simulink model "Didou_Telemetry"  (R2020a)
settings: Solver=FixedStepAuto  StartTime=0.0  StopTime=inf  RelTol=1e-3
libraries: robotlib x9
settings Model: SimulationMode=accelerator  Creator=alexemdesgagne  LastModifiedBy=alexemdesgagne
settings OptimizationCC: EnhancedBackFolding=on  PassReuseOutputArgsAs=Individual arguments  ZeroExternalMemoryAtStartup=off  ZeroInternalMemoryAtStartup=off  MaxStackSize=64  OptimizeBlockOrder=speed  DifferentSizesBufferReuse=on  OptimizationCustomize=off  EfficientTunableParamExpr=on
settings DebuggingCC: ParameterTunabilityLossMsg=error
settings HardwareCC: ProdBitPerPointer=32  ProdBitPerSizeT=32  ProdBitPerPtrDiffT=32  ProdLargestAtomicFloat=None  ProdIntDivRoundTo=Undefined  ProdEndianess=Unspecified  ProdWordSize=32  ProdHWDeviceType=Generic->Unspecified (assume 32-bit Generic)
settings SFSimCC: MATLABDynamicMemAlloc=off
settings RTWCC: SystemTargetFile=ert.tlc  HardwareBoard=Robot Operating System (ROS)  TemplateMakefile=ert_default_tmf  Toolchain=Catkin  TargetLang=C++
settings CodeAppCC: ForceParamTrailComments=on  IgnoreCustomStorageClasses=off  OperatorAnnotations=on  SimulinkDataObjDesc=on  SFDataObjDesc=on  InsertBlockDesc=on

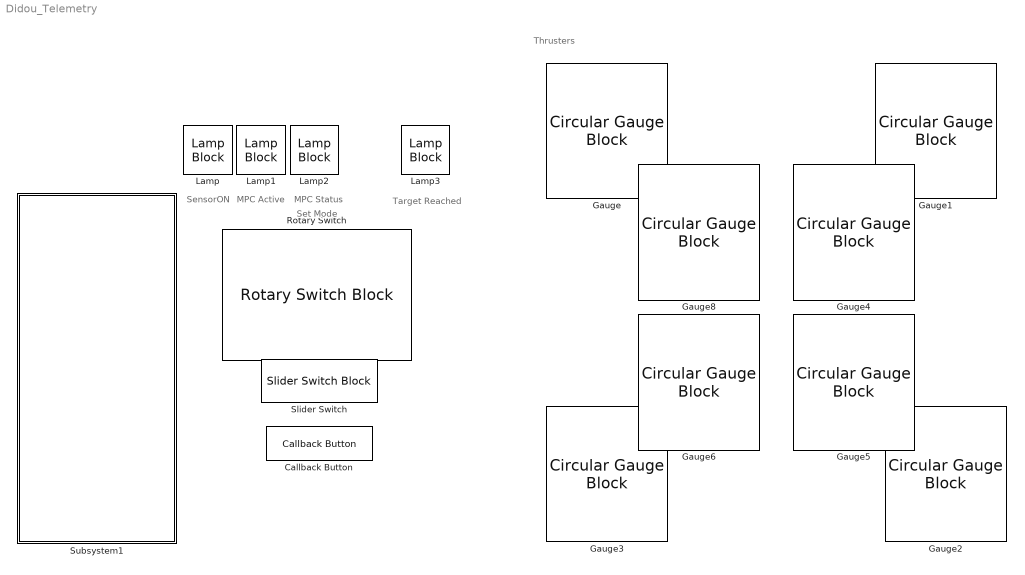
== system Didou_Telemetry ==
  note: Thrusters
  note: Target Reached
  note: MPC Active
  note: SensorON
  note: MPC Status
  note: Set Mode
  Callback Button : CallbackButton  ButtonText=Dry Test
      settings: ClickFcn=sim('dry_test', 60);
  Gauge{,1..6,8} (8 alike) : CircularGaugeBlock  ScaleMin=-40  ScaleMax=50
  Lamp{,1..3} (4 alike) : LampBlock  LabelPosition=Hide
  Rotary Switch : RotarySwitchBlock  LabelPosition=Hide
      settings: Values={{'MPC AUTO', 'MPC 3DMouse', '3DMouse model', '3DMouse B matrix', 'Soft Kill', 'MPC Single Wpts'}, [10 19 20 21 0 11]}
  Slider Switch : SliderSwitchBlock
      settings: Values={{'Off', 'On'}, [0 1]}
  Subsystem1 : Subsystem

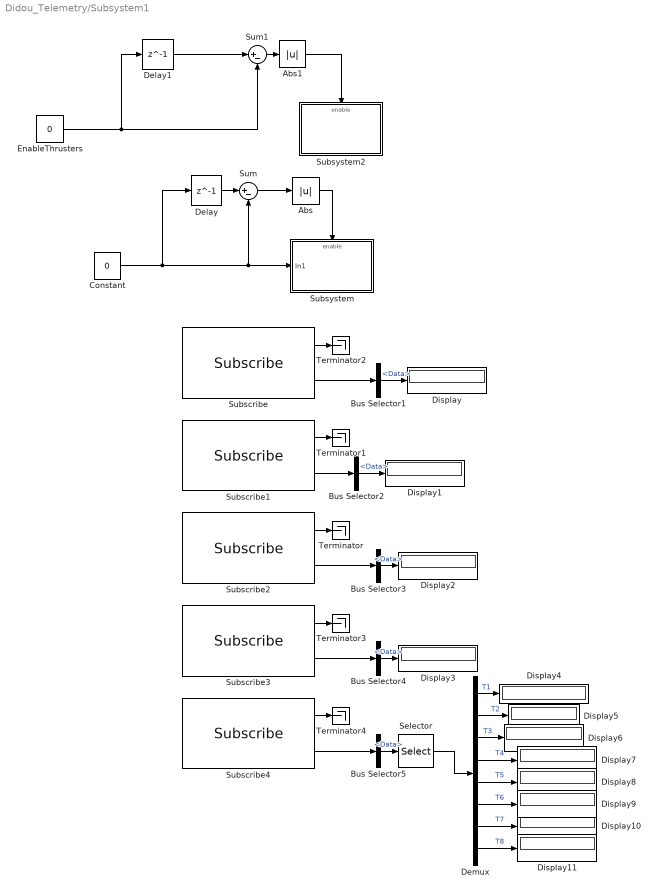
== system Didou_Telemetry/Subsystem1 ==
  Abs : Abs
  Abs1 : Abs
  Bus Selector{1..5} (5 alike) : BusSelector  OutputSignals=Data
  Constant : Constant  Value=0
  Delay : Delay  DelayLength=1
  Delay1 : Delay  DelayLength=1
  Demux : Demux  Outputs=8
  Display{,1..11} (12 alike) : Display
  EnableThrusters : Constant  Value=0
  Selector : Selector  InputPortWidth=128  IndexOptions=Index vector (dialog)  Indices=[1:8]  OutputSizes=1
  Subscribe : robotlib/Subscribe  topicSource=Select from ROS network  topic=/proc_control/sensor_on  messageType=std_msgs/Bool  sampleTime=-1  messageQueueLength=1
  Subscribe1 : robotlib/Subscribe  topicSource=Select from ROS network  topic=/proc_control/is_mpc_active  messageType=std_msgs/Bool  sampleTime=-1  messageQueueLength=1
  Subscribe2 : robotlib/Subscribe  topicSource=Select from ROS network  topic=/proc_control/mpc_status  messageType=std_msgs/Int8  sampleTime=-1  messageQueueLength=1
  Subscribe3 : robotlib/Subscribe  topicSource=Select from ROS network  topic=/proc_control/target_reached  messageType=std_msgs/Bool  sampleTime=-1  messageQueueLength=1
  Subscribe4 : robotlib/Subscribe  topicSource=Specify your own  topic=/telemetry/thruster_newton  messageType=std_msgs/Int8MultiArray  sampleTime=-1  messageQueueLength=1
  Subsystem : Subsystem
  Subsystem2 : Subsystem
  Sum : Sum  Inputs=|+-
  Sum1 : Sum  Inputs=|+-
  Terminator{,1..4} (5 alike) : Terminator
  wires:
  Subscribe/2 -> Bus Selector1/1
  Subscribe1/1 -> Terminator1/1
  Delay/1 -> Sum/1
  Subscribe/1 -> Terminator2/1
  Subscribe2/1 -> Terminator/1
  Bus Selector1/1 -> Display/1  "<Data>"
  Constant/1 -> Delay/1, Sum/2, Subsystem/1(In1)
  Subscribe2/2 -> Bus Selector3/1
  Bus Selector3/1 -> Display2/1  "<Data>"
  Subscribe1/2 -> Bus Selector2/1
  Sum/1 -> Abs/1
  Bus Selector2/1 -> Display1/1  "<Data>"
  Abs/1 -> Subsystem/Enable
  Sum1/1 -> Abs1/1
  Delay1/1 -> Sum1/1
  Abs1/1 -> Subsystem2/Enable
  EnableThrusters/1 -> Sum1/2, Delay1/1
  Subscribe3/1 -> Terminator3/1
  Bus Selector4/1 -> Display3/1  "<Data>"
  Subscribe3/2 -> Bus Selector4/1
  Subscribe4/2 -> Bus Selector5/1
  Subscribe4/1 -> Terminator4/1
  Demux/1 -> Display4/1  "T1"
  Demux/2 -> Display5/1  "T2"
  Demux/3 -> Display6/1  "T3"
  Demux/4 -> Display7/1  "T4"
  Demux/5 -> Display8/1  "T5"
  Demux/6 -> Display9/1  "T6"
  Demux/7 -> Display10/1  "T7"
  Demux/8 -> Display11/1  "T8"
  Bus Selector5/1 -> Selector/1  "<Data>"
  Selector/1 -> Demux/1

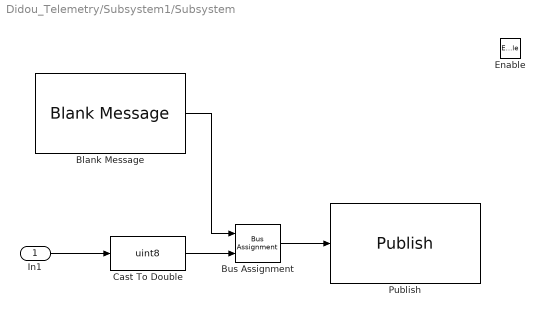
== system Didou_Telemetry/Subsystem1/Subsystem ==
  In1 : Inport
  Enable : EnablePort
  Blank Message : robotlib/Blank Message  messageClass=Message  entityType=std_msgs/UInt8  messageType=std_msgs/UInt8  SampleTime=inf
  Bus Assignment : BusAssignment  AssignedSignals=Data
  Cast To Double : DataTypeConversion  OutDataTypeStr=uint8
  Publish : robotlib/Publish  topicSource=Specify your own  topic=/proc_control/set_mode  messageType=std_msgs/UInt8  messageQueueLength=1
  wires:
  Blank Message/1 -> Bus Assignment/1
  In1/1 -> Cast To Double/1
  Bus Assignment/1 -> Publish/1
  Cast To Double/1 -> Bus Assignment/2

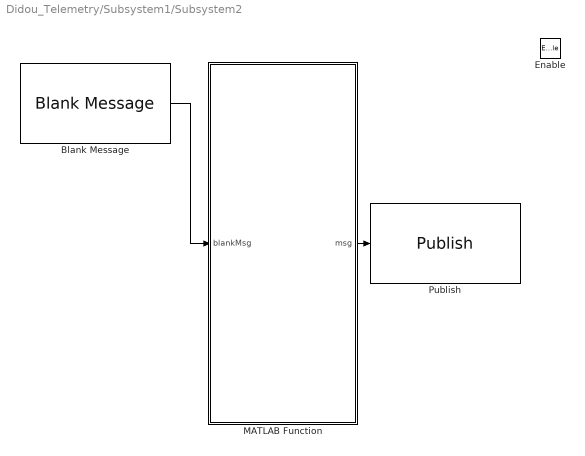
== system Didou_Telemetry/Subsystem1/Subsystem2 ==
  Enable : EnablePort
  Blank Message : robotlib/Blank Message  messageClass=Message  entityType=sonia_common/ActivateAllPS  messageType=sonia_common/ActivateAllPS  SampleTime=inf
  MATLAB Function : MATLAB Function  TreatAsAtomicUnit=on  SystemSampleTime=1/60
  Publish : robotlib/Publish  topicSource=Specify your own  topic=/provider_power/activate_all_ps  messageType=sonia_common/ActivateAllPS  messageQueueLength=1
  wires:
  Blank Message/1 -> MATLAB Function/1(blankMsg)
  MATLAB Function/1(msg) -> Publish/1

== matlab function Didou_Telemetry/Subsystem1/Subsystem2/MATLAB Function ==
  data: blankMsg input; msg output Bus: SL_Bus_Didou_Telemetry_sonia_common_ActivateAllPS
function msg = assignEnableThrusters(blankMsg)
% assignStringInput - Assign a string a ROS message to specified input string
%
% MSG = assignStringInput(blankMsg, STR) assigns the input string, STR, to
%  a string field in the ROS message, blankMsg, and outputs the updated
%  ROS message.
%
%  Inputs
%    blankMsg: A bus for a 'std_msgs/String' message. This is 
%        used to initialize the output.
%    str: An array of uint8 that will be assigned to the 'Data' field
%        in blankMsg. The entire array is assumed to be a valid sequence of
%        character ASCII values.
% 
%  Outputs:
%    msg: A bus for a 'std_msgs/String' message, with the 'Data'
%        field set to a string.

%   Copyright 2015 The MathWorks, Inc.
%#codegen

% Note: The datatype of 'msg' has been explicitly set to the appropriate 
% Simulink bus type ("Bus: SL_Bus_robotROSMessageUsageExample_std_msgs_String"). 
%
% If the model name is changed, the datatype needs to be changed as well:
%   1) Click "Edit Data" in the Editor toolstrip to open "Ports and Data Manager"
%   2) Select "msg". From the "Type" dropdown, select "--- Refresh data types ---"
%   3) Set datatype to "Bus: SL_Bus_<modelname>_std_msgs_String"
   
msg = blankMsg;
msg.Slave = uint8(49);
msg.Bus = uint8(0);
msg.Data = true;
